simulink model "gm_PID_Attitude_ver7_5"  (R2022a)
settings: Solver=FixedStepDiscrete  StartTime=0.0  StopTime=0.1  RelTol=1e-3
libraries: hdlmdlgenlib x2, simulink x1
settings Model: Creator=space  LastModifiedBy=space
settings OptimizationCC: BlockReduction=off  ConditionallyExecuteInputs=off  DefaultParameterBehavior=Inlined  InheritOutputTypeSmallerThanSingle=on
settings DebuggingCC: AlgebraicLoopMsg=error  ArtificialAlgebraicLoopMsg=none  InheritedTsInSrcMsg=none  SingleTaskRateTransMsg=error
settings HardwareCC: ProdBitPerPointer=32  ProdBitPerSizeT=32  ProdBitPerPtrDiffT=32  ProdLargestAtomicFloat=None  ProdIntDivRoundTo=Undefined  ProdEndianess=Unspecified  ProdWordSize=32  ProdHWDeviceType=ASIC/FPGA->ASIC/FPGA  TargetBitPerPointer=64  TargetBitPerSizeT=64  TargetBitPerPtrDiffT=64  TargetLongLongMode=on  TargetIntDivRoundTo=Zero  TargetEndianess=LittleEndian  TargetWordSize=64  TargetHWDeviceType=Custom Processor->MATLAB Host Computer  ProdEqTarget=off

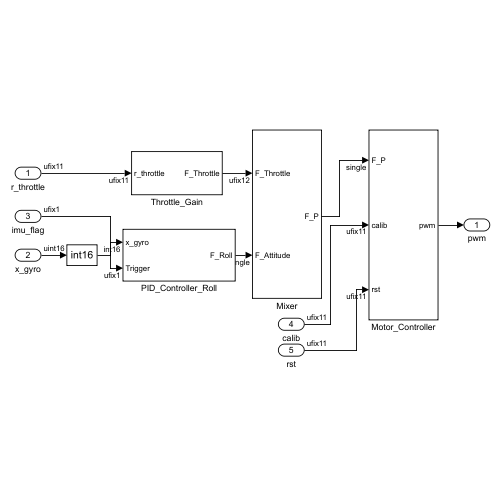
[thumbnail: Simulink's stored preview of the top-level diagram]
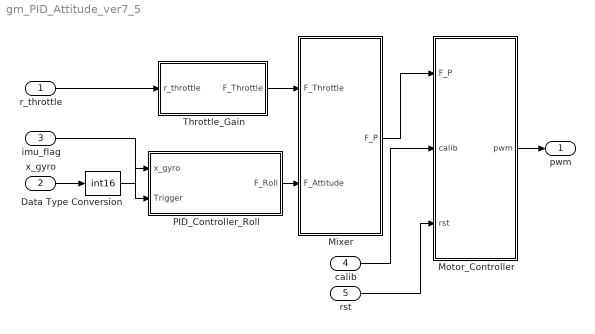
== system gm_PID_Attitude_ver7_5 ==
  r_throttle : Inport  OutDataTypeStr=fixdt(0, 11, 0)  PortDimensions=1  SampleTime=50000000
  x_gyro : Inport  Port=2  OutDataTypeStr=uint16  PortDimensions=1  SampleTime=50000000
  imu_flag : Inport  Port=3  OutDataTypeStr=fixdt(0, 1, 0)  PortDimensions=1  SampleTime=50000000
  calib : Inport  Port=4  OutDataTypeStr=fixdt(0, 11, 0)  PortDimensions=1  SampleTime=50000000
  rst : Inport  Port=5  OutDataTypeStr=fixdt(0, 11, 0)  PortDimensions=1  SampleTime=50000000
  Data Type Conversion : DataTypeConversion  OutDataTypeStr=int16  SaturateOnIntegerOverflow=off  RndMeth=Floor
  Mixer : Subsystem
  Motor_Controller : Subsystem
  PID_Controller_Roll : Subsystem
  Throttle_Gain : Subsystem
  pwm : Outport  SampleTime=50000000  VectorParamsAs1DForOutWhenUnconnected=off
  wires:
  r_throttle/1 -> Throttle_Gain/1(r_throttle)
  x_gyro/1 -> Data Type Conversion/1
  imu_flag/1 -> PID_Controller_Roll/2(Trigger)
  calib/1 -> Motor_Controller/2(calib)
  rst/1 -> Motor_Controller/3(rst)
  Data Type Conversion/1 -> PID_Controller_Roll/1(x_gyro)
  Mixer/1(F_P) -> Motor_Controller/1(F_P)
  Motor_Controller/1(pwm) -> pwm/1
  PID_Controller_Roll/1(F_Roll) -> Mixer/2(F_Attitude)
  Throttle_Gain/1(F_Throttle) -> Mixer/1(F_Throttle)

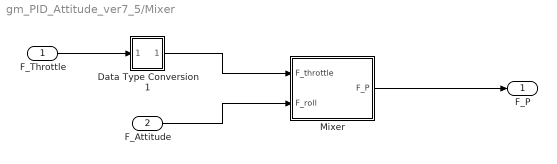
== system gm_PID_Attitude_ver7_5/Mixer ==
  F_Throttle : Inport  OutDataTypeStr=fixdt(0, 12, 0)  PortDimensions=1  SampleTime=50000000
  F_Attitude : Inport  Port=2  OutDataTypeStr=single  PortDimensions=1  SampleTime=50000000
  Data Type Conversion1 : Subsystem
      mask Display: disp('NFP\nconv');
  Mixer : Subsystem
  F_P : Outport  SampleTime=50000000
  wires:
  F_Throttle/1 -> Data Type Conversion1/1(In1)
  F_Attitude/1 -> Mixer/2(F_roll)
  Mixer/1(F_P) -> F_P/1
  Data Type Conversion1/1(Out1) -> Mixer/1(F_throttle)

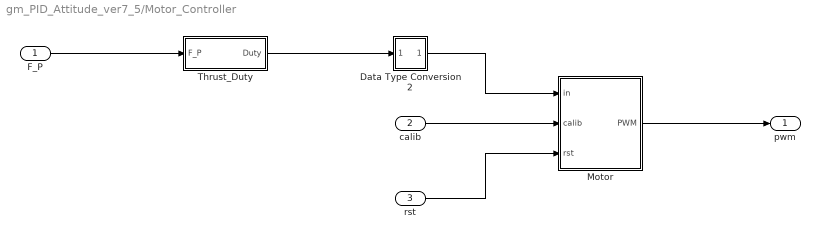
== system gm_PID_Attitude_ver7_5/Motor_Controller ==
  F_P : Inport  OutDataTypeStr=single  PortDimensions=1  SampleTime=50000000
  calib : Inport  Port=2  OutDataTypeStr=fixdt(0, 11, 0)  PortDimensions=1  SampleTime=50000000
  rst : Inport  Port=3  OutDataTypeStr=fixdt(0, 11, 0)  PortDimensions=1  SampleTime=50000000
  Data Type Conversion2 : Subsystem
      mask Display: disp('NFP\nconv');
  Motor : Subsystem
  Thrust_Duty : Subsystem
  pwm : Outport  SampleTime=50000000
  wires:
  F_P/1 -> Thrust_Duty/1(F_P)
  calib/1 -> Motor/2(calib)
  rst/1 -> Motor/3(rst)
  Motor/1(PWM) -> pwm/1
  Thrust_Duty/1(Duty) -> Data Type Conversion2/1(In1)
  Data Type Conversion2/1(Out1) -> Motor/1(in)

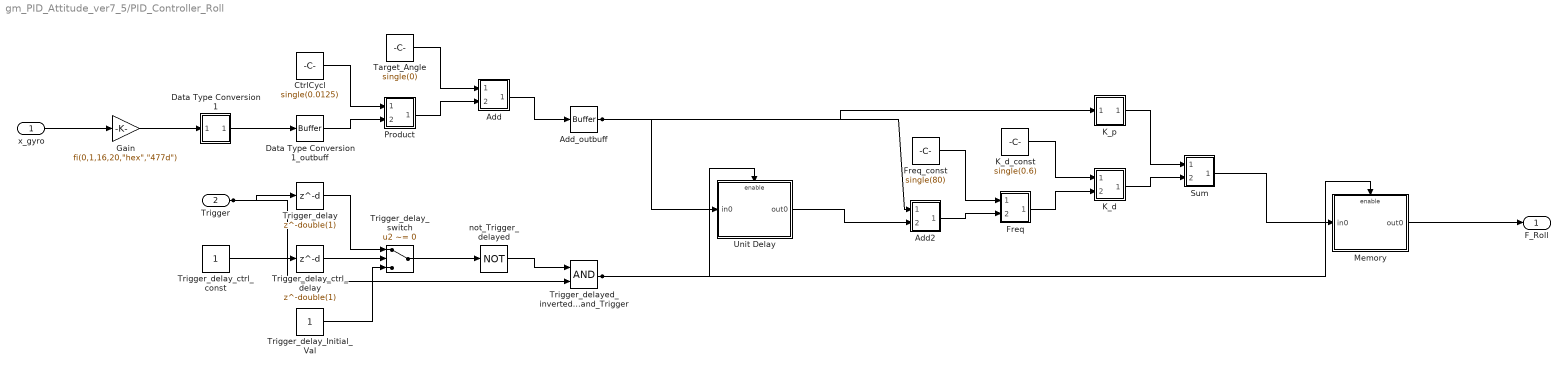
== system gm_PID_Attitude_ver7_5/PID_Controller_Roll ==
  x_gyro : Inport  OutDataTypeStr=int16  PortDimensions=1  SampleTime=50000000
  Trigger : Inport  Port=2  OutDataTypeStr=fixdt(0,1,0,'DataTypeOverride', 'Off')  SampleTime=50000000
  Add : Subsystem
      mask Display: disp('NFP\nadd');
  Add2 : Subsystem
      mask Display: disp('NFP\nadd');
  Add_outbuff : hdlmdlgenlib/Buffer
      settings: SourceProductBaseCode=SL
  CtrlCycl : Constant  Value=single(0.0125)  VectorParams1D=off  OutDataTypeStr=single  SampleTime=50000000
  Data Type Conversion1 : Subsystem
      mask Display: disp('NFP\nconv');
  Data Type Conversion1_outbuff : hdlmdlgenlib/Buffer
      settings: SourceProductBaseCode=SL
  Freq : Subsystem
      mask Display: disp('NFP\nmul');
  Freq_const : Constant  Value=single(80)  OutDataTypeStr=single  SampleTime=50000000
  Gain : Gain  Gain="fi(0,1,16,20,\"hex\",\"477d\")"  ParamDataTypeStr=fixdt(1, 16, 20)  OutDataTypeStr=fixdt(1, 32, 20)  SampleTime=50000000
  K_d : Subsystem
      mask Display: disp('NFP\nmul');
  K_d_const : Constant  Value=single(0.6)  OutDataTypeStr=single  SampleTime=50000000
  K_p : Subsystem
      mask Display: disp('NFP\ngain_pow2');
  Memory : Subsystem
      settings: MinAlgLoopOccurrences=on
  Product : Subsystem
      mask Display: disp('NFP\nmul');
  Sum : Subsystem
      mask Display: disp('NFP\nadd');
  Target_Angle : Constant  Value=single(0)  VectorParams1D=off  OutDataTypeStr=single  SampleTime=50000000
  Trigger_delay : Delay  DelayLength=double(1)  InitialCondition=0
  Trigger_delay_Initial_Val : Constant  OutDataTypeStr=fixdt(0, 1, 0)  SampleTime=50000000
  Trigger_delay_ctrl_const : Constant  OutDataTypeStr=boolean  SampleTime=50000000
  Trigger_delay_ctrl_delay : Delay  DelayLength=double(1)  InitialCondition=0
  Trigger_delay_switch : Switch  Criteria=u2 ~= 0  Threshold=double(0)  OutDataTypeStr=fixdt(0, 1, 0)  SampleTime=50000000  SaturateOnIntegerOverflow=off  InputSameDT=off
  Trigger_delayed_inverted_and_Trigger : Logic  AllPortsSameDT=off  OutDataTypeStr=fixdt(0, 1, 0)  SampleTime=50000000
  Unit Delay : Subsystem
      settings: MinAlgLoopOccurrences=on
  not_Trigger_delayed : Logic  Operator=NOT  Inputs=1  AllPortsSameDT=off  OutDataTypeStr=fixdt(0, 1, 0)  SampleTime=50000000
  F_Roll : Outport  SampleTime=50000000  InitialOutput=0
  wires:
  Trigger/1 -> Trigger_delayed_inverted_and_Trigger/2, Trigger_delay/1
  x_gyro/1 -> Gain/1
  Memory/1(out0) -> F_Roll/1
  Trigger_delay_switch/1 -> not_Trigger_delayed/1
  not_Trigger_delayed/1 -> Trigger_delayed_inverted_and_Trigger/1
  Trigger_delayed_inverted_and_Trigger/1 -> Unit Delay/Enable, Memory/Enable
  Trigger_delay/1 -> Trigger_delay_switch/1
  Trigger_delay_Initial_Val/1 -> Trigger_delay_switch/3
  Trigger_delay_ctrl_const/1 -> Trigger_delay_ctrl_delay/1
  Trigger_delay_ctrl_delay/1 -> Trigger_delay_switch/2
  Add_outbuff/1 -> Add2/1(In1), K_p/1(In1), Unit Delay/1(in0)
  Data Type Conversion1_outbuff/1 -> Product/2(In2)
  CtrlCycl/1 -> Product/1(In1)
  Gain/1 -> Data Type Conversion1/1(In1)
  Target_Angle/1 -> Add/1(In1)
  Unit Delay/1(out0) -> Add2/2(In2)
  Freq_const/1 -> Freq/1(In1)
  K_d_const/1 -> K_d/1(In1)
  K_p/1(Out1) -> Sum/1(In1)
  Add/1(Out1) -> Add_outbuff/1
  Add2/1(Out1) -> Freq/2(In2)
  Data Type Conversion1/1(Out1) -> Data Type Conversion1_outbuff/1
  Product/1(Out1) -> Add/2(In2)
  Sum/1(Out1) -> Memory/1(in0)
  Freq/1(Out1) -> K_d/2(In2)
  K_d/1(Out1) -> Sum/2(In2)

== system gm_PID_Attitude_ver7_5/Throttle_Gain ==
  r_throttle : Inport  OutDataTypeStr=fixdt(0, 11, 0)  PortDimensions=1  SampleTime=50000000
  Throttle_Gain : MATLAB Function  TreatAsAtomicUnit=on
  F_Throttle : Outport  SampleTime=50000000  VectorParamsAs1DForOutWhenUnconnected=off
  wires:
  r_throttle/1 -> Throttle_Gain/1(r_throttle)
  Throttle_Gain/1(F_Throttle) -> F_Throttle/1

== system gm_PID_Attitude_ver7_5/Mixer/Data Type Conversion1 ==
  In1 : Inport
  Data Type Conversion1 : DataTypeConversion  OutDataTypeStr=single  SampleTime=50000000  SaturateOnIntegerOverflow=off  RndMeth=Floor
  Out1 : Outport
  wires:
  In1/1 -> Data Type Conversion1/1
  Data Type Conversion1/1 -> Out1/1

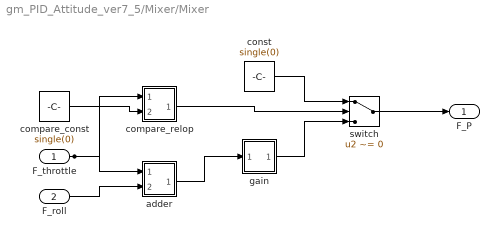
== system gm_PID_Attitude_ver7_5/Mixer/Mixer ==
  F_throttle : Inport  OutDataTypeStr=single  PortDimensions=1  SampleTime=50000000
  F_roll : Inport  Port=2  OutDataTypeStr=single  PortDimensions=1  SampleTime=50000000
  adder : Subsystem
      mask Display: disp('NFP\nadd');
  compare_const : Constant  Value=single(0)  OutDataTypeStr=single  SampleTime=50000000
  compare_relop : Subsystem
      mask Display: disp('NFP\nrelop');
  const : Constant  Value=single(0)  VectorParams1D=off  OutDataTypeStr=single  SampleTime=50000000
  gain : Subsystem
      mask Display: disp('NFP\ngain_pow2');
  switch : Switch  Criteria=u2 ~= 0  Threshold=double(0)  OutDataTypeStr=single  SampleTime=50000000  SaturateOnIntegerOverflow=off  InputSameDT=off
  F_P : Outport  SampleTime=50000000  VectorParamsAs1DForOutWhenUnconnected=off
  wires:
  F_throttle/1 -> adder/1(In1), compare_relop/1(In1)
  F_roll/1 -> adder/2(In2)
  switch/1 -> F_P/1
  const/1 -> switch/1
  compare_const/1 -> compare_relop/2(In2)
  gain/1(Out1) -> switch/3
  compare_relop/1(Out1) -> switch/2
  adder/1(Out1) -> gain/1(In1)

== system gm_PID_Attitude_ver7_5/Motor_Controller/Data Type Conversion2 ==
  In1 : Inport
  Data Type Conversion2 : DataTypeConversion  OutDataTypeStr=uint32  SampleTime=50000000  SaturateOnIntegerOverflow=off  RndMeth=Floor
  Out1 : Outport
  wires:
  In1/1 -> Data Type Conversion2/1
  Data Type Conversion2/1 -> Out1/1

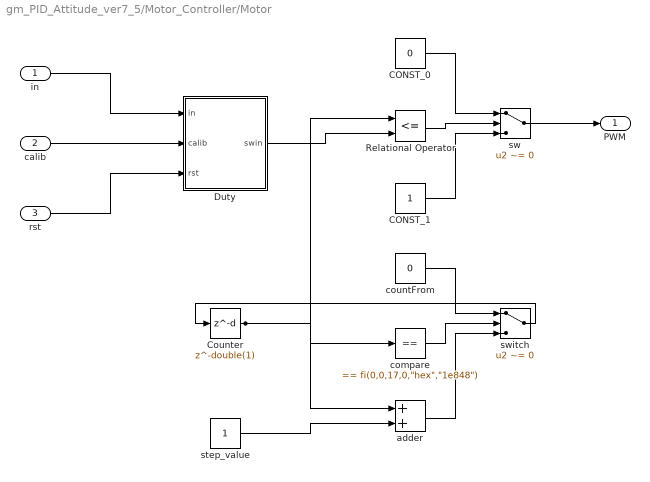
== system gm_PID_Attitude_ver7_5/Motor_Controller/Motor ==
  in : Inport  OutDataTypeStr=uint32  PortDimensions=1  SampleTime=50000000
  calib : Inport  Port=2  OutDataTypeStr=fixdt(0, 11, 0)  PortDimensions=1  SampleTime=50000000
  rst : Inport  Port=3  OutDataTypeStr=fixdt(0, 11, 0)  PortDimensions=1  SampleTime=50000000
  CONST_0 : Constant  Value=0  OutDataTypeStr=fixdt(0, 1, 0)  SampleTime=50000000
  CONST_1 : Constant  OutDataTypeStr=fixdt(0, 1, 0)  SampleTime=50000000
  Counter : Delay  DelayLength=double(1)  InitialCondition=0  SampleTime=50000000
  Duty : Subsystem
  Relational Operator : RelationalOperator  Operator=<=  OutDataTypeStr=boolean  SampleTime=50000000  InputSameDT=off
  adder : Sum  AccumDataTypeStr=fixdt(0, 17, 0)  OutDataTypeStr=fixdt(0, 17, 0)  SampleTime=50000000
  compare : simulink/Logic and Bit Operations/Compare To Constant  relop===  const="fi(0,0,17,0,\"hex\",\"1e848\")"  OutDataTypeStr=boolean
  countFrom : Constant  Value=0  VectorParams1D=off  OutDataTypeStr=fixdt(0, 17, 0)  SampleTime=50000000
  step_value : Constant  VectorParams1D=off  OutDataTypeStr=fixdt(0, 17, 0)  SampleTime=50000000
  sw : Switch  Criteria=u2 ~= 0  Threshold=double(0)  OutDataTypeStr=fixdt(0, 1, 0)  SampleTime=50000000  SaturateOnIntegerOverflow=off  InputSameDT=off
  switch : Switch  Criteria=u2 ~= 0  Threshold=double(0)  OutDataTypeStr=fixdt(0, 17, 0)  SampleTime=50000000  SaturateOnIntegerOverflow=off  InputSameDT=off
  PWM : Outport  SampleTime=50000000
  wires:
  in/1 -> Duty/1(in)
  calib/1 -> Duty/2(calib)
  rst/1 -> Duty/3(rst)
  CONST_0/1 -> sw/1
  CONST_1/1 -> sw/3
  Duty/1(swin) -> Relational Operator/2
  Relational Operator/1 -> sw/2
  sw/1 -> PWM/1
  Counter/1 -> compare/1, adder/1, Relational Operator/1
  adder/1 -> switch/3
  step_value/1 -> adder/2
  countFrom/1 -> switch/1
  switch/1 -> Counter/1
  compare/1 -> switch/2

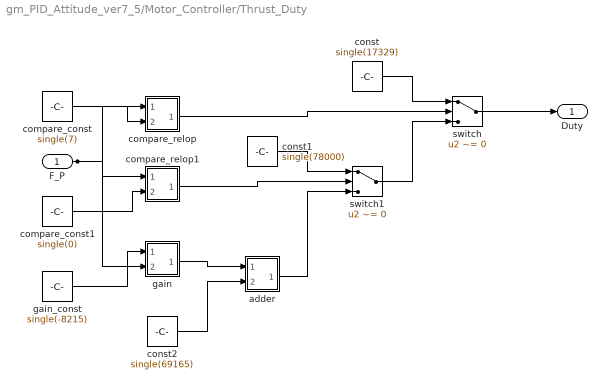
== system gm_PID_Attitude_ver7_5/Motor_Controller/Thrust_Duty ==
  F_P : Inport  OutDataTypeStr=single  PortDimensions=1  SampleTime=50000000
  adder : Subsystem
      mask Display: disp('NFP\nadd');
  compare_const : Constant  Value=single(7)  OutDataTypeStr=single  SampleTime=50000000
  compare_const1 : Constant  Value=single(0)  OutDataTypeStr=single  SampleTime=50000000
  compare_relop : Subsystem
      mask Display: disp('NFP\nrelop');
  compare_relop1 : Subsystem
      mask Display: disp('NFP\nrelop');
  const : Constant  Value=single(17329)  VectorParams1D=off  OutDataTypeStr=single  SampleTime=50000000
  const1 : Constant  Value=single(78000)  VectorParams1D=off  OutDataTypeStr=single  SampleTime=50000000
  const2 : Constant  Value=single(69165)  VectorParams1D=off  OutDataTypeStr=single  SampleTime=50000000
  gain : Subsystem
      mask Display: disp('NFP\nmul');
  gain_const : Constant  Value=single(-8215)  OutDataTypeStr=single  SampleTime=50000000
  switch : Switch  Criteria=u2 ~= 0  Threshold=double(0)  OutDataTypeStr=single  SampleTime=50000000  SaturateOnIntegerOverflow=off  InputSameDT=off
  switch1 : Switch  Criteria=u2 ~= 0  Threshold=double(0)  OutDataTypeStr=single  SampleTime=50000000  SaturateOnIntegerOverflow=off  InputSameDT=off
  Duty : Outport  SampleTime=50000000  VectorParamsAs1DForOutWhenUnconnected=off
  wires:
  F_P/1 -> gain/2(In2), compare_relop1/1(In1), compare_relop/1(In1)
  switch/1 -> Duty/1
  switch1/1 -> switch/3
  const/1 -> switch/1
  const1/1 -> switch1/1
  compare_const/1 -> compare_relop/2(In2)
  const2/1 -> adder/2(In2)
  compare_const1/1 -> compare_relop1/2(In2)
  gain_const/1 -> gain/1(In1)
  compare_relop/1(Out1) -> switch/2
  adder/1(Out1) -> switch1/3
  compare_relop1/1(Out1) -> switch1/2
  gain/1(Out1) -> adder/1(In1)

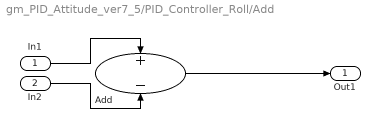
== system gm_PID_Attitude_ver7_5/PID_Controller_Roll/Add ==
  In1 : Inport
  In2 : Inport  Port=2
  Add : Sum  Inputs=+-  OutDataTypeStr=single  SampleTime=50000000
  Out1 : Outport
  wires:
  In1/1 -> Add/1
  In2/1 -> Add/2
  Add/1 -> Out1/1

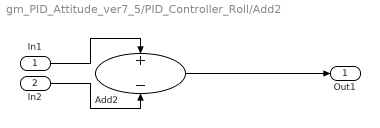
== system gm_PID_Attitude_ver7_5/PID_Controller_Roll/Add2 ==
  In1 : Inport
  In2 : Inport  Port=2
  Add2 : Sum  Inputs=+-  OutDataTypeStr=single  SampleTime=50000000
  Out1 : Outport
  wires:
  In1/1 -> Add2/1
  In2/1 -> Add2/2
  Add2/1 -> Out1/1

== system gm_PID_Attitude_ver7_5/PID_Controller_Roll/Data Type Conversion1 ==
  In1 : Inport
  Data Type Conversion1 : DataTypeConversion  OutDataTypeStr=single  SampleTime=50000000  SaturateOnIntegerOverflow=off  RndMeth=Floor
  Out1 : Outport
  wires:
  In1/1 -> Data Type Conversion1/1
  Data Type Conversion1/1 -> Out1/1

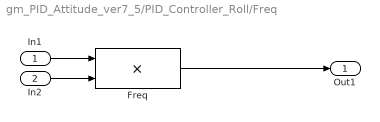
== system gm_PID_Attitude_ver7_5/PID_Controller_Roll/Freq ==
  In1 : Inport
  In2 : Inport  Port=2
  Freq : Product  Inputs=**  OutDataTypeStr=single  SampleTime=50000000
  Out1 : Outport
  wires:
  In1/1 -> Freq/1
  In2/1 -> Freq/2
  Freq/1 -> Out1/1

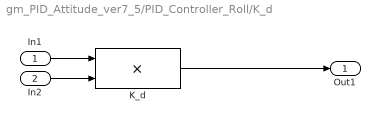
== system gm_PID_Attitude_ver7_5/PID_Controller_Roll/K_d ==
  In1 : Inport
  In2 : Inport  Port=2
  K_d : Product  Inputs=**  OutDataTypeStr=single  SampleTime=50000000
  Out1 : Outport
  wires:
  In1/1 -> K_d/1
  In2/1 -> K_d/2
  K_d/1 -> Out1/1

== system gm_PID_Attitude_ver7_5/PID_Controller_Roll/K_p ==
  In1 : Inport
  K_p : Gain  Gain=single(0.5)
  Out1 : Outport
  wires:
  In1/1 -> K_p/1
  K_p/1 -> Out1/1

== system gm_PID_Attitude_ver7_5/PID_Controller_Roll/Memory ==
  in0 : Inport  OutDataTypeStr=single  SampleTime=50000000
  Trigger_emulated : EnablePort  OutDataTypeStr=fixdt(0,1,0,'DataTypeOverride', 'Off')
  Memory : UnitDelay  InitialCondition=double(0)  SampleTime=50000000
  out0 : Outport  OutDataTypeStr=single  SampleTime=50000000  InitialOutput=0
  wires:
  Memory/1 -> out0/1
  in0/1 -> Memory/1

== system gm_PID_Attitude_ver7_5/PID_Controller_Roll/Product ==
  In1 : Inport
  In2 : Inport  Port=2
  Product : Product  Inputs=**  OutDataTypeStr=single  SampleTime=50000000
  Out1 : Outport
  wires:
  In1/1 -> Product/1
  In2/1 -> Product/2
  Product/1 -> Out1/1

== system gm_PID_Attitude_ver7_5/PID_Controller_Roll/Sum ==
  In1 : Inport
  In2 : Inport  Port=2
  Sum : Sum  OutDataTypeStr=single  SampleTime=50000000
  Out1 : Outport
  wires:
  In1/1 -> Sum/1
  In2/1 -> Sum/2
  Sum/1 -> Out1/1

== system gm_PID_Attitude_ver7_5/PID_Controller_Roll/Unit Delay ==
  in0 : Inport  OutDataTypeStr=single  SampleTime=50000000
  Trigger_emulated : EnablePort  OutDataTypeStr=fixdt(0,1,0,'DataTypeOverride', 'Off')
  Unit Delay : UnitDelay  InitialCondition=single(0)  SampleTime=50000000
  out0 : Outport  OutDataTypeStr=single  SampleTime=50000000  InitialOutput=0
  wires:
  Unit Delay/1 -> out0/1
  in0/1 -> Unit Delay/1

== system gm_PID_Attitude_ver7_5/Mixer/Mixer/adder ==
  In1 : Inport
  In2 : Inport  Port=2
  adder : Sum  OutDataTypeStr=single  SampleTime=50000000
  Out1 : Outport
  wires:
  In1/1 -> adder/1
  In2/1 -> adder/2
  adder/1 -> Out1/1

== system gm_PID_Attitude_ver7_5/Mixer/Mixer/compare_relop ==
  In1 : Inport
  In2 : Inport  Port=2
  compare_relop : RelationalOperator  Operator===  OutDataTypeStr=boolean  SampleTime=50000000
  Out1 : Outport
  wires:
  In1/1 -> compare_relop/1
  In2/1 -> compare_relop/2
  compare_relop/1 -> Out1/1

== system gm_PID_Attitude_ver7_5/Mixer/Mixer/gain ==
  In1 : Inport
  gain : Gain  Gain=single(0.25)
  Out1 : Outport
  wires:
  In1/1 -> gain/1
  gain/1 -> Out1/1

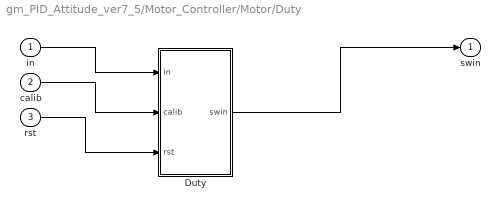
== system gm_PID_Attitude_ver7_5/Motor_Controller/Motor/Duty ==
  in : Inport  OutDataTypeStr=uint32  PortDimensions=1  SampleTime=50000000
  calib : Inport  Port=2  OutDataTypeStr=fixdt(0, 11, 0)  PortDimensions=1  SampleTime=50000000
  rst : Inport  Port=3  OutDataTypeStr=fixdt(0, 11, 0)  PortDimensions=1  SampleTime=50000000
  Duty : MATLAB Function  TreatAsAtomicUnit=on
  swin : Outport  SampleTime=50000000  VectorParamsAs1DForOutWhenUnconnected=off
  wires:
  in/1 -> Duty/1(in)
  calib/1 -> Duty/2(calib)
  rst/1 -> Duty/3(rst)
  Duty/1(swin) -> swin/1

== system gm_PID_Attitude_ver7_5/Motor_Controller/Thrust_Duty/adder ==
  In1 : Inport
  In2 : Inport  Port=2
  adder : Sum  OutDataTypeStr=single  SampleTime=50000000
  Out1 : Outport
  wires:
  In1/1 -> adder/1
  In2/1 -> adder/2
  adder/1 -> Out1/1

== system gm_PID_Attitude_ver7_5/Motor_Controller/Thrust_Duty/compare_relop ==
  In1 : Inport
  In2 : Inport  Port=2
  compare_relop : RelationalOperator  Operator=>  OutDataTypeStr=boolean  SampleTime=50000000
  Out1 : Outport
  wires:
  In1/1 -> compare_relop/1
  In2/1 -> compare_relop/2
  compare_relop/1 -> Out1/1

== system gm_PID_Attitude_ver7_5/Motor_Controller/Thrust_Duty/compare_relop1 ==
  In1 : Inport
  In2 : Inport  Port=2
  compare_relop1 : RelationalOperator  Operator=<=  OutDataTypeStr=boolean  SampleTime=50000000
  Out1 : Outport
  wires:
  In1/1 -> compare_relop1/1
  In2/1 -> compare_relop1/2
  compare_relop1/1 -> Out1/1

== system gm_PID_Attitude_ver7_5/Motor_Controller/Thrust_Duty/gain ==
  In1 : Inport
  In2 : Inport  Port=2
  gain : Product  Inputs=**  OutDataTypeStr=single  SampleTime=50000000
  Out1 : Outport
  wires:
  In1/1 -> gain/1
  In2/1 -> gain/2
  gain/1 -> Out1/1

== matlab function gm_PID_Attitude_ver7_5/Motor_Controller/Motor/Duty/Duty ==
  settings: fimath=fimath('RoundingMethod', 'Floor','OverflowAction', 'Wrap','ProductMode', 'FullPrecision', 'SumMode', 'FullPrecision')
  data: in input; swin output; calib input; rst input
function swin = Duty(in, calib, rst)

if rst > 1000
    %reset
    rst = 0x1E848u32;
    swin = rst;
    %swin = [rst; rst; rst; rst];
elseif calib > 1050
    %PWM -> MAX
    max = 0x1F4u32;
    swin = max;
    %swin = [max; max; max; max];
elseif calib == 1024
    %PWM -> MIN
    min = 0x130B0u32;
    swin = min;
    %swin = [min; min; min; min];
elseif calib < 1000
    %PWM -> thrust
    swin = in;
    %swin = [in(1); in(2); in(3); in(4)];
else
    err = 0x130B0u32;
    swin = err;
    %swin = [err; err; err; err];
end

== matlab function gm_PID_Attitude_ver7_5/Throttle_Gain/Throttle_Gain ==
  settings: fimath=fimath('RoundingMethod', 'Floor','OverflowAction', 'Wrap','ProductMode', 'FullPrecision', 'SumMode', 'FullPrecision')
  data: F_Throttle output; r_throttle input
function F_Throttle = Throttle_Gain(r_throttle)

F_Throttle = r_throttle / 56 - 44 / 7;
